simulink model "WaermepumpeGrundlageIch"  (R2013a)
settings: Solver=ode4  StartTime=0.0  StopTime=inf  RelTol=1e-3
libraries: Thermolib x74, simulink x2
(part 1 of 2)
settings Model: Creator=studi  LastModifiedBy=Admin
settings DataIOCC: SignalLoggingSaveFormat=ModelDataLogs
settings DebuggingCC: MultiTaskDSMMsg=warning  MultiTaskCondExecSysMsg=none  StrictBusMsg=None
settings RTWCC: IncludeERTFirstTime=on
settings GRTTargetCC: CodeReplacementLibrary=None  CPPClassGenCompliant=on

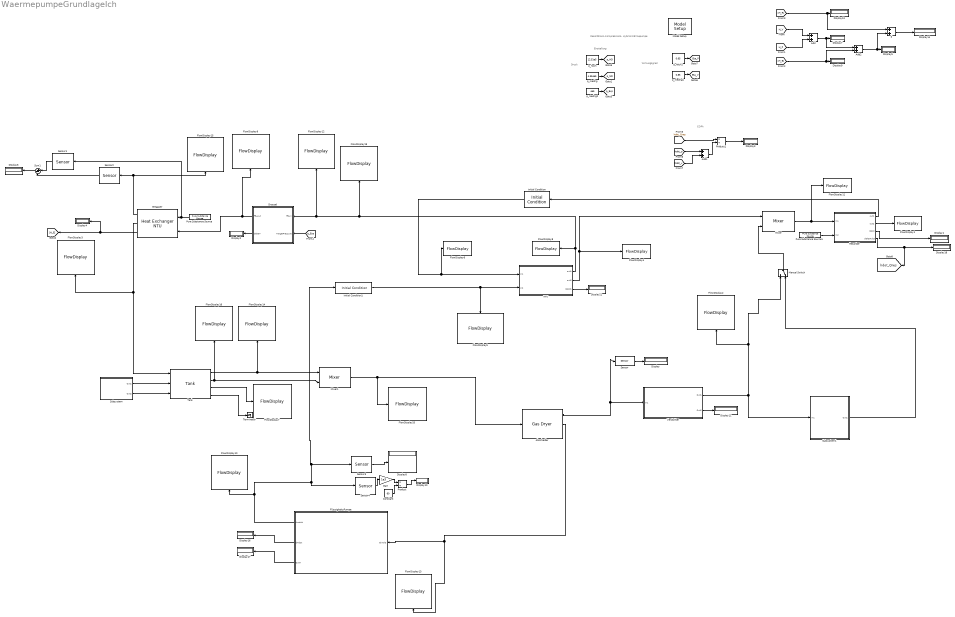
== system WaermepumpeGrundlageIch ==
  note: Resorbtions-Kompressions-
      | Hybrid-Wärmepumpe
  note: Einstellung
  note: Druck
  note: Wirkungsgrad
  note: COPh
  Abscheider : Thermolib/Components/Heat and Mass Transfer/Gas Dryer  Abscheid_eff=[0.4 1]  ndots=[0 5]  P_Loss=[0,1e3]  show_pf_ports=off  show_info_port=on  default_order_in_ports={'in','PFin'}  default_order_out_ports={'out','liquid','PFout','info'}
  Add : Sum
  Add1 : Sum
  Add2 : Sum
  Constant : Constant  Value=60
  Display{,1..11,13..14,16..18,21} (18 alike) : Display
  Drossel : Subsystem
      mask help: Jawooohl
      mask Help: Looking for help??
      mask Display:
      | fprintf('Isenthalp')
      | port_label('input', 1, 'in');
      | port_label('input', 2, 'p_target');
      | port_label('output', 1, 'out');
      | port_label('output', 2, '\Delta T','texmode','on');
  Entgaser : Thermolib/Components/Heat and Mass Transfer/Heat Exchanger NTU  selection=Counter Flow  show_UA_port=off  UA_Overall=3000  T_initial=273+20  A_env=1  T_env=273+25  k_env=0  p_loss_1=[0,1e3]  p_loss_2=[0,1e3]  thermal_mass=1  UA_flow1_mass1=0  UA_flow2_mass2=0  show_pf_ports=off  show_info_port=off  default_order_in_ports={'in1','in2','PFin1','PFin2'}  default_order_out_ports={'out1','out2','Qdot','PFout1','PFout2','info'}
  FlowDisplay1 : Thermolib/Sinks/FlowDisplay  bus_type=FlowBus  mdot=off kg/s  m_unit=mg  ndot=off mol/s  n_unit=mmol  temperature=on  T_unit=Celsius  pressure=on  p_unit=Pa  enthalpy=off  Hdot_unit=W  H_unit=mJ  entropy=off  Sdot_unit=W/K  S_unit=mJ/K  gibbs_energy=off  Gdot_unit=W  G_unit=mJ  heat_capacity=off  Cpdot_unit=W/K  Cp_unit=mJ/K  energy_content=off  U_unit=mW/K  vapor_fraction=off  molar_fraction=off  flag=0.8152
  FlowDisplay10 : Thermolib/Sinks/FlowDisplay  bus_type=FlowBus  mdot=off kg/s  m_unit=mg  ndot=on mol/s  n_unit=mmol  temperature=on  T_unit=Kelvin  pressure=on  p_unit=bar  enthalpy=on  Hdot_unit=W  H_unit=mJ  entropy=off  Sdot_unit=W/K  S_unit=mJ/K  gibbs_energy=off  Gdot_unit=W  G_unit=mJ  heat_capacity=off  Cpdot_unit=W/K  Cp_unit=mJ/K  energy_content=off  U_unit=mW/K  vapor_fraction=on  molar_fraction=on  flag=0.1812
  FlowDisplay11 : Thermolib/Sinks/FlowDisplay  bus_type=FlowBus  mdot=off kg/s  m_unit=mg  ndot=off mol/s  n_unit=mmol  temperature=on  T_unit=Celsius  pressure=on  p_unit=Pa  enthalpy=off  Hdot_unit=W  H_unit=mJ  entropy=off  Sdot_unit=W/K  S_unit=mJ/K  gibbs_energy=off  Gdot_unit=W  G_unit=mJ  heat_capacity=off  Cpdot_unit=W/K  Cp_unit=mJ/K  energy_content=off  U_unit=mW/K  vapor_fraction=off  molar_fraction=off  flag=0.1282
  FlowDisplay12 : Thermolib/Sinks/FlowDisplay  bus_type=FlowBus  mdot=off kg/s  m_unit=mg  ndot=off mol/s  n_unit=mmol  temperature=on  T_unit=Celsius  pressure=on  p_unit=bar  enthalpy=off  Hdot_unit=W  H_unit=mJ  entropy=off  Sdot_unit=W/K  S_unit=mJ/K  gibbs_energy=off  Gdot_unit=W  G_unit=mJ  heat_capacity=off  Cpdot_unit=W/K  Cp_unit=mJ/K  energy_content=off  U_unit=mW/K  vapor_fraction=off  molar_fraction=off  flag=0.5199
  FlowDisplay13 : Thermolib/Sinks/FlowDisplay  bus_type=FlowBus  mdot=off kg/s  m_unit=mg  ndot=on mol/s  n_unit=mmol  temperature=on  T_unit=Kelvin  pressure=on  p_unit=bar  enthalpy=on  Hdot_unit=W  H_unit=mJ  entropy=off  Sdot_unit=W/K  S_unit=mJ/K  gibbs_energy=off  Gdot_unit=W  G_unit=mJ  heat_capacity=off  Cpdot_unit=W/K  Cp_unit=mJ/K  energy_content=off  U_unit=mW/K  vapor_fraction=on  molar_fraction=on  flag=0.9645
  FlowDisplay14 : Thermolib/Sinks/FlowDisplay  bus_type=FlowBus  mdot=off kg/s  m_unit=mg  ndot=off mol/s  n_unit=mmol  temperature=on  T_unit=Celsius  pressure=on  p_unit=bar  enthalpy=off  Hdot_unit=W  H_unit=mJ  entropy=off  Sdot_unit=W/K  S_unit=mJ/K  gibbs_energy=off  Gdot_unit=W  G_unit=mJ  heat_capacity=off  Cpdot_unit=W/K  Cp_unit=mJ/K  energy_content=off  U_unit=mW/K  vapor_fraction=off  molar_fraction=off  flag=0.9654
  FlowDisplay15 : Thermolib/Sinks/FlowDisplay  bus_type=FlowBus  mdot=on kg/s  m_unit=mg  ndot=on mol/s  n_unit=mmol  temperature=on  T_unit=Kelvin  pressure=on  p_unit=bar  enthalpy=on  Hdot_unit=W  H_unit=mJ  entropy=off  Sdot_unit=W/K  S_unit=mJ/K  gibbs_energy=off  Gdot_unit=W  G_unit=mJ  heat_capacity=on  Cpdot_unit=W/K  Cp_unit=mJ/K  energy_content=off  U_unit=mW/K  vapor_fraction=on  molar_fraction=on  flag=0.8000
  FlowDisplay16 : Thermolib/Sinks/FlowDisplay  bus_type=FlowBus  mdot=off kg/s  m_unit=mg  ndot=off mol/s  n_unit=mmol  temperature=on  T_unit=Celsius  pressure=on  p_unit=bar  enthalpy=off  Hdot_unit=W  H_unit=mJ  entropy=off  Sdot_unit=W/K  S_unit=mJ/K  gibbs_energy=off  Gdot_unit=W  G_unit=mJ  heat_capacity=off  Cpdot_unit=W/K  Cp_unit=mJ/K  energy_content=off  U_unit=mW/K  vapor_fraction=off  molar_fraction=off  flag=0.3184
  FlowDisplay19 : Thermolib/Sinks/FlowDisplay  bus_type=FlowBus  mdot=off kg/s  m_unit=mg  ndot=on mol/s  n_unit=mmol  temperature=on  T_unit=Kelvin  pressure=on  p_unit=bar  enthalpy=on  Hdot_unit=W  H_unit=mJ  entropy=off  Sdot_unit=W/K  S_unit=mJ/K  gibbs_energy=off  Gdot_unit=W  G_unit=mJ  heat_capacity=off  Cpdot_unit=W/K  Cp_unit=mJ/K  energy_content=off  U_unit=mW/K  vapor_fraction=on  molar_fraction=on  flag=0.3878
  FlowDisplay2 : Thermolib/Sinks/FlowDisplay  bus_type=FlowBus  mdot=off kg/s  m_unit=mg  ndot=on mol/s  n_unit=mmol  temperature=on  T_unit=Celsius  pressure=on  p_unit=bar  enthalpy=on  Hdot_unit=W  H_unit=mJ  entropy=off  Sdot_unit=W/K  S_unit=mJ/K  gibbs_energy=off  Gdot_unit=W  G_unit=mJ  heat_capacity=off  Cpdot_unit=W/K  Cp_unit=mJ/K  energy_content=off  U_unit=mW/K  vapor_fraction=on  molar_fraction=on  flag=0.7145
  FlowDisplay20 : Thermolib/Sinks/FlowDisplay  bus_type=StateBus  mdot=on kg/s  m_unit=kg  ndot=off mol/s  n_unit=mol  temperature=on  T_unit=Celsius  pressure=on  p_unit=bar  enthalpy=on  Hdot_unit=W  H_unit=J  entropy=off  Sdot_unit=W/K  S_unit=mJ/K  gibbs_energy=off  Gdot_unit=W  G_unit=mJ  heat_capacity=off  Cpdot_unit=W/K  Cp_unit=mJ/K  energy_content=off  U_unit=mW/K  vapor_fraction=on  molar_fraction=on  flag=0.8658
  FlowDisplay3 : Thermolib/Sinks/FlowDisplay  bus_type=FlowBus  mdot=off kg/s  m_unit=mg  ndot=off mol/s  n_unit=mmol  temperature=on  T_unit=Celsius  pressure=on  p_unit=bar  enthalpy=off  Hdot_unit=W  H_unit=mJ  entropy=off  Sdot_unit=W/K  S_unit=mJ/K  gibbs_energy=off  Gdot_unit=W  G_unit=mJ  heat_capacity=off  Cpdot_unit=W/K  Cp_unit=mJ/K  energy_content=off  U_unit=mW/K  vapor_fraction=off  molar_fraction=off  flag=0.0870
  FlowDisplay4 : Thermolib/Sinks/FlowDisplay  bus_type=FlowBus  mdot=off kg/s  m_unit=mg  ndot=off mol/s  n_unit=mmol  temperature=on  T_unit=Kelvin  pressure=on  p_unit=Pa  enthalpy=off  Hdot_unit=W  H_unit=mJ  entropy=off  Sdot_unit=W/K  S_unit=mJ/K  gibbs_energy=off  Gdot_unit=W  G_unit=mJ  heat_capacity=off  Cpdot_unit=W/K  Cp_unit=mJ/K  energy_content=off  U_unit=mW/K  vapor_fraction=off  molar_fraction=off  flag=0.2788
  FlowDisplay5 : Thermolib/Sinks/FlowDisplay  bus_type=FlowBus  mdot=off kg/s  m_unit=mg  ndot=off mol/s  n_unit=mmol  temperature=on  T_unit=Kelvin  pressure=on  p_unit=Pa  enthalpy=off  Hdot_unit=W  H_unit=mJ  entropy=off  Sdot_unit=W/K  S_unit=mJ/K  gibbs_energy=off  Gdot_unit=W  G_unit=mJ  heat_capacity=off  Cpdot_unit=W/K  Cp_unit=mJ/K  energy_content=off  U_unit=mW/K  vapor_fraction=off  molar_fraction=off  flag=0.0144
  FlowDisplay6 : Thermolib/Sinks/FlowDisplay  bus_type=FlowBus  mdot=off kg/s  m_unit=mg  ndot=off mol/s  n_unit=mmol  temperature=on  T_unit=Kelvin  pressure=on  p_unit=Pa  enthalpy=off  Hdot_unit=W  H_unit=mJ  entropy=off  Sdot_unit=W/K  S_unit=mJ/K  gibbs_energy=off  Gdot_unit=W  G_unit=mJ  heat_capacity=off  Cpdot_unit=W/K  Cp_unit=mJ/K  energy_content=off  U_unit=mW/K  vapor_fraction=off  molar_fraction=off  flag=0.8314
  FlowDisplay7 : Thermolib/Sinks/FlowDisplay  bus_type=StateBus  mdot=on kg/s  m_unit=kg  ndot=off mol/s  n_unit=mol  temperature=on  T_unit=Celsius  pressure=on  p_unit=bar  enthalpy=on  Hdot_unit=W  H_unit=J  entropy=off  Sdot_unit=W/K  S_unit=mJ/K  gibbs_energy=off  Gdot_unit=W  G_unit=mJ  heat_capacity=off  Cpdot_unit=W/K  Cp_unit=mJ/K  energy_content=off  U_unit=mW/K  vapor_fraction=on  molar_fraction=on  flag=0.6126
  FlowDisplay8 : Thermolib/Sinks/FlowDisplay  bus_type=FlowBus  mdot=off kg/s  m_unit=mg  ndot=off mol/s  n_unit=mmol  temperature=on  T_unit=Kelvin  pressure=on  p_unit=Pa  enthalpy=off  Hdot_unit=W  H_unit=mJ  entropy=off  Sdot_unit=W/K  S_unit=mJ/K  gibbs_energy=off  Gdot_unit=W  G_unit=mJ  heat_capacity=off  Cpdot_unit=W/K  Cp_unit=mJ/K  energy_content=off  U_unit=mW/K  vapor_fraction=off  molar_fraction=off  flag=0.0312
  FlowDisplay9 : Thermolib/Sinks/FlowDisplay  bus_type=FlowBus  mdot=off kg/s  m_unit=mg  ndot=off mol/s  n_unit=mmol  temperature=on  T_unit=Celsius  pressure=on  p_unit=bar  enthalpy=off  Hdot_unit=W  H_unit=mJ  entropy=off  Sdot_unit=W/K  S_unit=mJ/K  gibbs_energy=off  Gdot_unit=W  G_unit=mJ  heat_capacity=off  Cpdot_unit=W/K  Cp_unit=mJ/K  energy_content=off  U_unit=mW/K  vapor_fraction=off  molar_fraction=off  flag=0.5216
  FlüssigkeitsPumpe : Subsystem
      mask Display:
      | path=pwd;
      | path_n=cat(2,pwd,'\Pumpe.PNG');
      | image(path_n);
      | port_label('input', 1, 'In');
      | port_label('output', 1, 'Out');
      | port_label('output', 3, 'Eta_p');
      | port_label('output', 2, 'dh');
  Gain : Gain  Gain=1e3
  IWU : Subsystem  mask(Heat Exchanger NTU){selection=Counter Flow, show_UA_port=off, UA_Overall=100, T_initial=273+20, A_env=1, T_env=273+20, k_env=0, p_loss_1=[0,1e1], p_loss_2=[0,1e1], thermal_mass=1, UA_flow1_mass1=0, UA_flow2_mass2=0, show_pf_ports=off, show_info_port=off, default_order_in_ports={'in1','in2','PFin1','PFin2'}, default_order_out_ports={'out1','out2','Qdot','PFout1','PFout2','info'}}
      mask prompts: selection "Flow direction:"; show_UA_port "Overall heat exchange coefficient from external"; UA_Overall "Coefficient of overall heat transfer rate [W/K]:"; T_initial "Initial temperature [K]:"; A_env "Total surface to environment  [m^2]:"; T_env "Environment temperature [K]:"; k_env "Coefficient for calculating heat exchange with the environment [W / m2 K]:"; p_loss_1 "Pressure loss factor [Pa/(g/s) 2] and minimum downstream pressure [Pa] for first flow:"; p_loss_2 "Pressure loss factor [Pa/(g/s) 2] and minimum downstream pressure [Pa] for second flow:"; thermal_mass "Thermal mass of the heat exchanger [Joules/K]:"; UA_flow1_mass1 "Coefficient of heat transfer rate from flow 1 to thermal mass 1 [W/K]"; UA_flow2_mass2 "Coefficient of heat transfer rate from flow 2 to thermal mass 2 [W/K]"; show_pf_ports "Show pressure feedback ports"; show_info_port "Show info port"
      mask help:
      | The Heat Exchanger block calculates the change of state of two media caused by indirect heat exchange. Three types of exchange are supported: counter flow, parallel flow and cross flow.
      |
      | The NTU-Method (number of transfer unit), used to model the heat exchanger, calculates the maximum possible heat transfer between the two flows. The actual heat transfer rate can be determined by calculating the effectiveness, which is the actual heat transfer divided by the maximum possible heat transfer.
      |
      | To model the thermal dynamics the input flows are passed through two thermal mass elements.
      mask init:
      | set_param(gcb, 'MaskSelfModifiable', 'on');
      | 
      | if selection==3
      |   icon = imread('heat_ex_pa.tif','tif');
      | end
      | if selection==1
      |   icon = imread('heat_ex_co.tif','tif');
      | end
      | if selection==2
      |   icon = imread('heat_ex_cr.tif','tif');
      | end
      | 
      | blk = gcb;
      | ioc = zeros(1,6);
      | 
      | ioc(1) = th_ShowPorts(blk,'PFin1','show_pf_ports','in','built-in/Constant',{'Value','0'});
      | ioc(2) = th_ShowPorts(blk,'PFin2','show_pf_ports','in','built-in/Constant',{'Value','0'});
      | ioc(3) = th_ShowPorts(blk,'UA','show_UA_port','in','built-in/Constant',{'Value','UA_Overall'});
      | ioc(4) = th_ShowPorts(blk,'PFout1','show_pf_ports','out','built-in/Terminator');
      | ioc(5) = th_ShowPorts(blk,'PFout2','show_pf_ports','out','built-in/Terminator');
      | ioc(6) = th_ShowPorts(blk,'info','show_info_port','out','built-in/Terminator');
      | 
      | if any(ioc)
      | 	base_draw_cmd = 'image(icon,[0.2,0.1,0.6,0.8])';
      | 	th_AddPortsToDrawingCmd(blk,base_draw_cmd)
      | end
      mask Help: eval('th_StartBlockHelp(gcb)');
      mask TypeOptions selection: Counter Flow | Cross Flow | Parallel Flow
      mask Callback show_UA_port:
      | a = {'on','on','on','on','on','on','on','on','on','on','on','on','on','on','off','off'};
      | b = {'on','on','off','on','on','on','on','on','on','on','on','on','on','on','off','off'};
      | 
      | 
      | 
      | switch get_param(gcb, 'show_UA_port')
      |     case 'on'
      |         set_param(gcb,'MaskVisibilities',	[b] );
      |     case 'off'
      |         set_param(gcb,'MaskVisibilities',	[a]);
      | end
      mask Display:
      | image(icon,[0.2,0.1,0.6,0.8])
      | port_label('output',1,'out1')
      | port_label('output',2,'out2')
      | port_label('output',3,'Qdot')
      | port_label('input',1,'in1')
      | port_label('input',2,'in2')
  Initial Condition : Thermolib/Miscellaneous/Initial Condition  disp_str=fprintf('Initial conditions:\n T = 298.15 [K]\np = 100000 [Pa]')  T=298.15 C  T_in=25  p=100000 bar  p_in=1  psi=[0.3 0.7]  species_local={'H2O', 'NH3'}  psi_local=[0.3 0.7]  use_fb=on  ndot=1 mol/s  ndot_in=0  switch_flow_type=1  flow_type=Molar Flow  Hdot=-117669.870695777  Sdot=156.374582351195  Gdot=-164292.952423785  Cpdot=48.0782778924394  x=[0.0658877601640708;0.956663479644059]  show_pf_ports=off  default_order_in_ports=off  default_order_out_ports=off
  Initial Condition1 : Thermolib/Miscellaneous/Initial Condition  disp_str=fprintf('Initial conditions:\n T = 298.15 [K]\np = 100000 [Pa]')  T=298.15 C  T_in=25  p=100000 bar  p_in=1  psi=[0.3 0.7]  species_local={'H2O', 'NH3'}  psi_local=[0.3 0.7]  use_fb=on  ndot=1 mol/s  ndot_in=0  switch_flow_type=1  flow_type=Molar Flow  Hdot=-117669.870695777  Sdot=156.374582351195  Gdot=-164292.952423785  Cpdot=48.0782778924394  x=[0.0658877601640708;0.956663479644059]  show_pf_ports=off  default_order_in_ports=off  default_order_out_ports=off
  Manual Switch : ManualSwitch  CurrentSetting=0
  Mixer : Thermolib/Components/Hydraulic/Mixer  Mode=mixer  P_Loss=[0,0.01e5]  p_out_method=p_out = weighted_mean(p1_in;p2_in)  default_order_in_ports={'in1','in2','ratio','PFin'}  default_order_out_ports={'out','in2 ','PFout1','PFout2','info'}  show_pf_ports=off  show_info_port=off
  Mixer1 : Thermolib/Components/Hydraulic/Mixer  Mode=mixer  P_Loss=[0,0.01e5]  p_out_method=p_out = weighted_mean(p1_in;p2_in)  default_order_in_ports={'in1','in2','ratio','PFin'}  default_order_out_ports={'out','in2 ','PFout1','PFout2','info'}  show_pf_ports=off  show_info_port=off
  Model Setup : Thermolib/Setup/Model Setup  starttime=10  endtime=20  loadWS=on  loadWSCommand=fc_LoadWorkspace  media_file=ChemicalMediaData.mat  constants_file=Constants.mat  species_reduced={'H2O', 'NH3'}  load_model_command=load ComponentData.mat  gas_eos_method=1  gas_mixing_rule=0  species_allow_liquid=[1 1]  species_allow_vapor=[1 1]  last_saved_thermolib_version=5.1.2.5490  liquid_eos_method=1  density_calculation_mode=0
  Product : Product  Inputs=*/
  Product1 : Product  Inputs=*/
  Pure Substance Source : Thermolib/Sources/Pure Substance Source  disp_str=fprintf('H2O Mass flow')  flow_type=Mass flow  switch_flow_type=3  ndot=1002 kg/s  ndot_in=1.002  T=313.15 K  T_in=273.15+40  p=100000 Pa  p_in=1e+5  T_p_x_switch=2  x=1e-005  species_local={'H2O'}  psi_local=1  psi=[1 0]
  Pure Substance Source1 : Thermolib/Sources/Pure Substance Source  disp_str=fprintf('H2O Mass flow')  flow_type=Mass flow  switch_flow_type=3  ndot=1000 kg/s  ndot_in=1  T=313.15 K  T_in=273.15+40  p=100000 Pa  p_in=1e+5  T_p_x_switch=2  x=1e-005  species_local={'H2O'}  psi_local=1  psi=[1 0]
  Resorber : Subsystem  AncestorBlock=Thermolib/Components/Heat and Mass Transfer/Heat Exchanger NTU  mask(Heat Exchanger NTU){selection=Counter Flow, show_UA_port=off, UA_Overall=3000, T_initial=273+20, A_env=0, T_env=273+20, k_env=0, p_loss_1=[0,1e3], p_loss_2=[0,1e3], thermal_mass=0.1, UA_flow1_mass1=0, UA_flow2_mass2=0, show_pf_ports=off, show_info_port=off, default_order_in_ports={'in1','in2','PFin1','PFin2'}, default_order_out_ports={'out1','out2','Qdot','PFout1','PFout2','info'}}
      mask prompts: selection "Flow direction:"; show_UA_port "Overall heat exchange coefficient from external"; UA_Overall "Coefficient of overall heat transfer rate [W/K]:"; T_initial "Initial temperature [K]:"; A_env "Total surface to environment  [m^2]:"; T_env "Environment temperature [K]:"; k_env "Coefficient for calculating heat exchange with the environment [W / m2 K]:"; p_loss_1 "Pressure loss factor [Pa/(g/s) 2] and minimum downstream pressure [Pa] for first flow:"; p_loss_2 "Pressure loss factor [Pa/(g/s) 2] and minimum downstream pressure [Pa] for second flow:"; thermal_mass "Thermal mass of the heat exchanger [Joules/K]:"; UA_flow1_mass1 "Coefficient of heat transfer rate from flow 1 to thermal mass 1 [W/K]"; UA_flow2_mass2 "Coefficient of heat transfer rate from flow 2 to thermal mass 2 [W/K]"; show_pf_ports "Show pressure feedback ports"; show_info_port "Show info port"
      mask help:
      | The Heat Exchanger block calculates the change of state of two media caused by indirect heat exchange. Three types of exchange are supported: counter flow, parallel flow and cross flow.
      |
      | The NTU-Method (number of transfer unit), used to model the heat exchanger, calculates the maximum possible heat transfer between the two flows. The actual heat transfer rate can be determined by calculating the effectiveness, which is the actual heat transfer divided by the maximum possible heat transfer.
      |
      | To model the thermal dynamics the input flows are passed through two thermal mass elements.
      mask init: same as WaermepumpeGrundlageIch/IWU
      mask Help: eval('th_StartBlockHelp(gcb)');
      mask TypeOptions selection: Counter Flow | Cross Flow | Parallel Flow
      mask Callback show_UA_port:
      | a = {'on','on','on','on','on','on','on','on','on','on','on','on','on','on','off','off'};
      | b = {'on','on','off','on','on','on','on','on','on','on','on','on','on','on','off','off'};
      | 
      | 
      | 
      | switch get_param(gcb, 'show_UA_port')
      |     case 'on'
      |         set_param(gcb,'MaskVisibilities',	[b] );
      |     case 'off'
      |         set_param(gcb,'MaskVisibilities',	[a]);
      | end
      mask Display:
      | image(icon,[0.2,0.1,0.6,0.8])
      | port_label('output',1,'out1')
      | port_label('output',2,'out2')
      | port_label('output',3,'Qdot')
      | port_label('output',4,'deltaHdot')
      | port_label('input',1,'in1')
      | port_label('input',2,'in2')
  S : Sum
  Sensor : Thermolib/Miscellaneous/Sensor  lst_physical_value=vdot_gas measured in m^3/h;  mult_fac=3600  add_fac=0  selected_signals=14
  Sensor1 : Thermolib/Miscellaneous/Sensor  lst_physical_value=Hdot measured in W;  mult_fac=1  add_fac=0  selected_signals=4
  Sensor2 : Thermolib/Miscellaneous/Sensor  lst_physical_value=Hdot measured in W;  mult_fac=1  add_fac=0  selected_signals=4
  Sensor3 : Thermolib/Miscellaneous/Sensor  lst_physical_value=vdot_gas measured in m^3/h;vdot_liquid measured in m^3/h;mdot measured in kg/s;psi H2O measured in -;  mult_fac=[3600 3600 0.001 1]  add_fac=[0 0 0 0]  selected_signals=[14 16 13 11]
  Sensor4 : Thermolib/Miscellaneous/Sensor  lst_physical_value=vdot_liquid measured in m^3/h;  mult_fac=3600  add_fac=0  selected_signals=16
  Subsystem : Subsystem  mask{m=0, a1=0, a2=0}
      mask prompts: m "Massenstrom"; a1 "Wasser Anteil"; a2 "Ammoniak Anteil"
      mask Display: fprintf('Massenstromregler')
  Subsystem1 : Subsystem
      mask Display:
      | path=pwd;
      | path_n=cat(2,pwd,'\Abscheider.png');
      | image(path_n);
  Sum1 : Sum  Inputs=|+-
  Tank : Thermolib/Components/Tanks/Tank  Volume=0.1  T_init=273+25  p_init=4e5  psi_init=[0.3 0.7]  p_min=1e4  mdot_out_method1=m.out = external  mdot_out_method2=m.out = external  species_local={'H2O', 'NH3'}  psi_local=[0.3 0.7]  x_init=0.3  mdot_out_pf_max=1000  mdot_out_pf_initial=1  mdot_out_pf_relaxation=0.3  show_pfout1_port=off  show_pfout2_port=off  Generic_Tank_radiobutton=off  Adiabatic_Tank_radiobutton=on  Isothermal_Tank_radiobutton=off  show_in1_port=on  show_in2_port=off  show_out1_port=on  show_out2_port=on  show_mdot_out1_port=on  show_mdot_out2_port=on  show_pfin1_port=off  show_pfin2_port=off  default_order_in_ports={'in1','in2','mdot_out1','mdot_out2','Qdot','PFin1','PFin2'}  default_order_out_ports={'out1','out2','state',' Qdot','PFout1','PFout2','info'}  T_p_x_switch=3  position_out1=1  position_out2=0  show_info_port=on
  Terminator : Terminator
  Verdichter : Subsystem  Description=Verdichter (Selbstgemacht)  mask(Verdichter Selfmade){}
      mask help: Polytrop
      mask Help: Frag Anton
      mask Display:
      | path=pwd;
      | path_n=cat(2,pwd,'\Verdichter.PNG');
      | image(path_n);
      | port_label('input', 1, 'In');
      | port_label('output', 1, 'Out');
      | port_label('output', 2,'\Delta Hdot','texmode','on');
  p_hoch : Constant  Value=12.51e5
  p_hoch1 : Constant  Value=0.65
  p_niedrig : Constant  Value=4.354e5
  p_niedrig1 : Constant  Value=0.85
  p_niedrig2 : Constant  Value=4e5
  tag scope: Eta_P=global, Eta_V=global, hdot_Qres=global, p_Exp=global, p_HD=global, p_ND=global
  wires:
  Abscheider/2 -> FlowDisplay13/1, FlüssigkeitsPumpe/1(Eintritt)
  Pure Substance Source/1 -> Sensor1/1, Entgaser/1
  [p_Exp] -> Drossel/2(TargetPressure)
  Resorber/2(out2) -> FlowDisplay1/1
  Resorber/3(Qdot) -> Display1/1
  Entgaser/3 -> Display4/1, [H_E]
  Drossel/1(FB_out) -> FlowDisplay9/1, Entgaser/2
  Drossel/2(deltaT) -> Display2/1
  [H_V] -> Add/1
  [H_P] -> Add/2
  Add/1 -> Add2/1, Display7/1
  [H_E] -> Add2/2, Display9/1
  Resorber/1(out1) -> Initial Condition/1
  Mixer/1 -> FlowDisplay11/1, Resorber/1(in1)
  [H_R] -> S/1, Display13/1
  Add2/1 -> S/2, Display5/1
  S/1 -> Display14/1
  Tank/1 -> FlowDisplay14/1, Mixer1/1
  Tank/2 -> Mixer1/2, FlowDisplay16/1
  p_hoch/1 -> [p_HD]
  p_niedrig/1 -> [p_ND]
  p_hoch1/1 -> [Eta_P]
  p_niedrig1/1 -> [Eta_V]
  Entgaser/2 -> FlowDisplay3/1, Tank/1
  Tank/3 -> FlowDisplay7/1
  IWU/2(out2) -> FlowDisplay4/1, Mixer/1
  IWU/1(out1) -> Drossel/1(FB_in), FlowDisplay12/1, FlowDisplay19/1, FlowDisplay8/1
  Initial Condition/1 -> FlowDisplay6/1, IWU/1(in1)
  IWU/3(Qdot1) -> Display21/1
  Tank/4 -> Terminator/1
  ? -> ?
  Abscheider/1 -> Sensor/1, Verdichter/1(In1)
  FlüssigkeitsPumpe/1("Austritt ") -> FlowDisplay10/1, Initial Condition1/1, Sensor3/1, Sensor4/1
  FlüssigkeitsPumpe/2("dHdot ") -> Display16/1
  FlüssigkeitsPumpe/3(Out4) -> Display17/1
  Initial Condition1/1 -> FlowDisplay5/1, IWU/2(in2)
  Sensor/1 -> Display/1
  Mixer1/1 -> FlowDisplay20/1, Abscheider/1
  Sensor3/1 -> Display8/1
  Product/1 -> Display10/1
  Constant/1 -> Product/2
  Sensor4/1 -> Gain/1
  Gain/1 -> Product/1
  Pure Substance Source1/1 -> Resorber/2(in2)
  Entgaser/1 -> Sensor2/1, FlowDisplay15/1
  p_niedrig2/1 -> [p_Exp]
  Sensor1/1 -> Sum1/1
  Sensor2/1 -> Sum1/2
  Sum1/1 -> Display6/1
  Verdichter/2(Out2) -> Display11/1
  Resorber/4(deltaHdot) -> [hdot_Qres], Display18/1
  Subsystem/1(Out1) -> Tank/2
  Subsystem/2(Out2) -> Tank/3
  [hdot_Qres] -> Product1/1
  [hdot_p] -> Add1/1
  [hdot_v] -> Add1/2
  Add1/1 -> Product1/2
  Product1/1 -> Display3/1
  Manual Switch/1 -> Mixer/2
  Verdichter/1(Out1) -> Subsystem1/1(In1), FlowDisplay2/1, Manual Switch/1
  Subsystem1/1(Out1) -> Manual Switch/2

== system WaermepumpeGrundlageIch/Drossel ==
  FB_in : Inport
  TargetPressure : Inport  Port=2
  Bus Assignment3 : BusAssignment  AssignedSignals=p
  Bus Selector5 : BusSelector  OutputSignals=p
  H-p-State : Thermolib/Thermodynamic States and Properties/H-p-State with Heat Exchange  k=0  A_total=0  T_env=273+20  relaxation_factor=0.01  conv_limit=0.1  hm_conv_limit=TH_THERM_H_P_STATE_HM_CONV_LIMIT  n_iteration=TH_THERM_H_P_STATE_NUM_ITER_MAX  T_initial=273+20  H_initial=0  ndot_zero_eps=1e-9
  MinMax : MinMax  Inputs=2
  Subtract : Sum  Inputs=+-
  T1 : BusSelector  OutputSignals=T
  T2 : BusSelector  OutputSignals=T
  Terminator3 : Terminator
  Terminator4 : Terminator
  FB_out : Outport
  deltaT : Outport  Port=2
  wires:
  H-p-State/1 -> T2/1, FB_out/1
  H-p-State/3 -> Terminator4/1
  H-p-State/2 -> Terminator3/1
  Bus Assignment3/1 -> H-p-State/1
  FB_in/1 -> T1/1, Bus Assignment3/1, Bus Selector5/1
  Bus Selector5/1 -> MinMax/1  "<p>"
  TargetPressure/1 -> MinMax/2
  MinMax/1 -> Bus Assignment3/2
  T1/1 -> Subtract/1  "<T>"
  T2/1 -> Subtract/2  "<T>"
  Subtract/1 -> deltaT/1

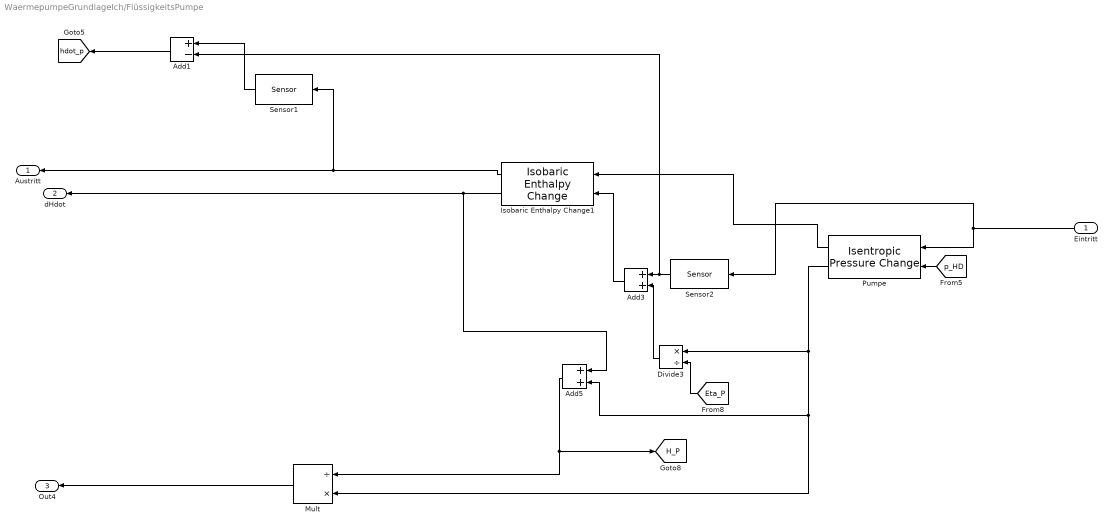
== system WaermepumpeGrundlageIch/FlüssigkeitsPumpe ==
  Eintritt : Inport
  Add1 : Sum  Inputs=+-
  Add3 : Sum
  Add5 : Sum
  Divide3 : Product  Inputs=*/
  Isobaric Enthalpy Change1 : Thermolib/Thermodynamic State Changes/Isobaric Enthalpy Change
  Mult : Product  Inputs=/*
  Pumpe : Thermolib/Thermodynamic State Changes/Isentropic Pressure Change
  Sensor1 : Thermolib/Miscellaneous/Sensor  lst_physical_value=Hdot measured in W;  mult_fac=1  add_fac=0  selected_signals=4
  Sensor2 : Thermolib/Miscellaneous/Sensor  lst_physical_value=Hdot measured in W;  mult_fac=1  add_fac=0  selected_signals=4
  "Austritt " : Outport
  "dHdot " : Outport  Port=2
  Out4 : Outport  Port=3
  tag scope: H_P=global, hdot_p=global
  wires:
  Eintritt/1 -> Pumpe/1, Sensor2/1
  Pumpe/2 -> Mult/2, Add5/2, Divide3/1
  [p_HD] -> Pumpe/2
  Pumpe/1 -> Isobaric Enthalpy Change1/1
  [Eta_P] -> Divide3/2
  Sensor2/1 -> Add1/2, Add3/1
  Divide3/1 -> Add3/2
  Add3/1 -> Isobaric Enthalpy Change1/2
  Isobaric Enthalpy Change1/2 -> Add5/1, "dHdot "/1
  Mult/1 -> Out4/1
  Add5/1 -> Mult/1, [H_P]
  Isobaric Enthalpy Change1/1 -> Sensor1/1, "Austritt "/1
  Add1/1 -> [hdot_p]
  Sensor1/1 -> Add1/1

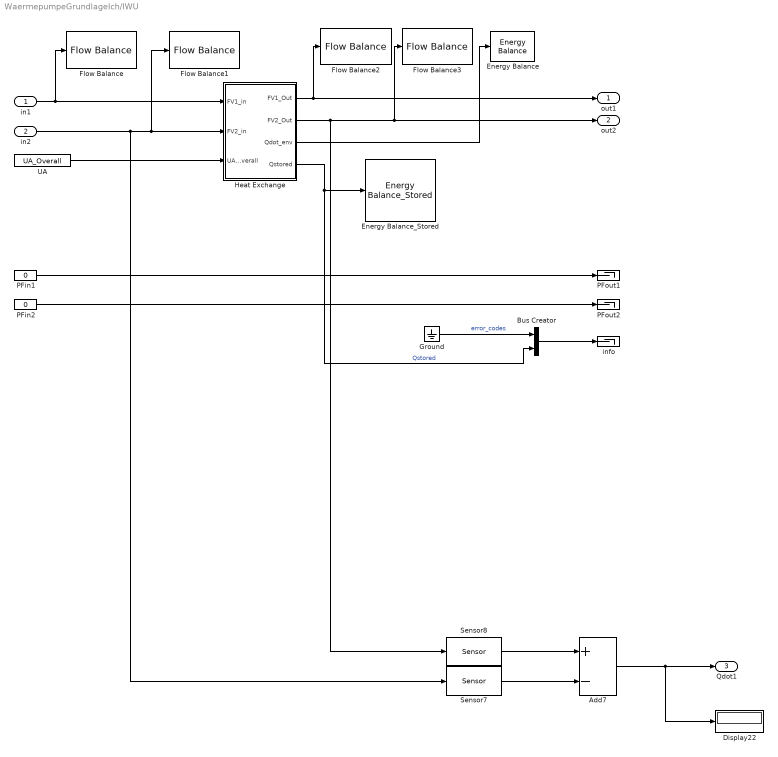
== system WaermepumpeGrundlageIch/IWU ==
  in1 : Inport
  in2 : Inport  Port=2
  Add7 : Sum  Inputs=+-
  Bus Creator : BusCreator  Inputs=2
  Display22 : Display
  Energy Balance : Thermolib/Balance/Energy Balance  asklabel=Use name of parent system  mainlabel=Thermolib/Components/Heat and Mass Transfer/Heat Exchanger NTU  label='Qdot environment'
  Energy Balance_Stored : Thermolib/Balance/Energy Balance_Stored  asklabel=Use name of parent system  mainlabel=Thermolib/Components/Heat and Mass Transfer/Heat Exchanger NTU  label='thermal mass energy'
  Flow Balance : Thermolib/Balance/Flow Balance  asklabel=Use name of parent system  mainlabel='Name here'  direction=in  label='In1'
  Flow Balance1 : Thermolib/Balance/Flow Balance  asklabel=Use name of parent system  mainlabel='Name here'  direction=in  label='in2'
  Flow Balance2 : Thermolib/Balance/Flow Balance  asklabel=Use name of parent system  mainlabel='Name here'  direction=out  label='out1'
  Flow Balance3 : Thermolib/Balance/Flow Balance  asklabel=Use name of parent system  mainlabel='Name here'  direction=out  label='out2'
  Ground : Ground
  Heat Exchange : Subsystem  TreatAsAtomicUnit=on
  PFin1 : Constant  Value=0
  PFin2 : Constant  Value=0
  PFout1 : Terminator
  PFout2 : Terminator
  Sensor7 : Thermolib/Miscellaneous/Sensor  lst_physical_value=Hdot measured in W;  mult_fac=1  add_fac=0  selected_signals=4
  Sensor8 : Thermolib/Miscellaneous/Sensor  lst_physical_value=Hdot measured in W;  mult_fac=1  add_fac=0  selected_signals=4
  UA : Constant  Value=UA_Overall
  info : Terminator
  out1 : Outport
  out2 : Outport  Port=2
  Qdot1 : Outport  Port=3
  wires:
  Ground/1 -> Bus Creator/1  "error_codes"
  Bus Creator/1 -> info/1
  Heat Exchange/4(Qstored) -> Bus Creator/2, Energy Balance_Stored/1  "Qstored"
  Heat Exchange/3(Qdot_env) -> Energy Balance/1
  Heat Exchange/1(FV1_Out) -> Flow Balance2/1, out1/1
  in1/1 -> Heat Exchange/1(FV1_in), Flow Balance/1
  PFin1/1 -> PFout1/1
  PFin2/1 -> PFout2/1
  UA/1 -> Heat Exchange/3(UA_overall)
  Heat Exchange/2(FV2_Out) -> Sensor8/1, Flow Balance3/1, out2/1
  in2/1 -> Sensor7/1, Flow Balance1/1, Heat Exchange/2(FV2_in)
  Sensor7/1 -> Add7/2
  Sensor8/1 -> Add7/1
  Add7/1 -> Qdot1/1, Display22/1

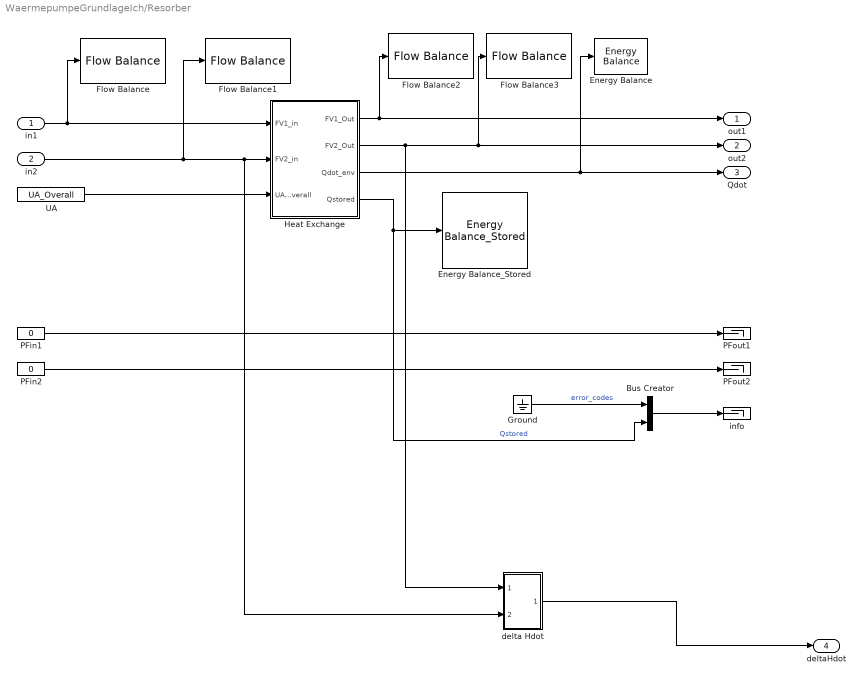
== system WaermepumpeGrundlageIch/Resorber ==
  in1 : Inport
  in2 : Inport  Port=2
  Bus Creator : BusCreator  Inputs=2
  Energy Balance : Thermolib/Balance/Energy Balance  asklabel=Use name of parent system  mainlabel=Thermolib/Components/Heat and Mass Transfer/Heat Exchanger NTU  label='Qdot environment'
  Energy Balance_Stored : Thermolib/Balance/Energy Balance_Stored  asklabel=Use name of parent system  mainlabel=Thermolib/Components/Heat and Mass Transfer/Heat Exchanger NTU  label='thermal mass energy'
  Flow Balance : Thermolib/Balance/Flow Balance  asklabel=Use name of parent system  mainlabel='Name here'  direction=in  label='In1'
  Flow Balance1 : Thermolib/Balance/Flow Balance  asklabel=Use name of parent system  mainlabel='Name here'  direction=in  label='in2'
  Flow Balance2 : Thermolib/Balance/Flow Balance  asklabel=Use name of parent system  mainlabel='Name here'  direction=out  label='out1'
  Flow Balance3 : Thermolib/Balance/Flow Balance  asklabel=Use name of parent system  mainlabel='Name here'  direction=out  label='out2'
  Ground : Ground
  Heat Exchange : Subsystem  TreatAsAtomicUnit=on
  PFin1 : Constant  Value=0
  PFin2 : Constant  Value=0
  PFout1 : Terminator
  PFout2 : Terminator
  UA : Constant  Value=UA_Overall
  delta Hdot : Subsystem
  info : Terminator
  out1 : Outport
  out2 : Outport  Port=2
  Qdot : Outport  Port=3
  deltaHdot : Outport  Port=4
  wires:
  UA/1 -> Heat Exchange/3(UA_overall)
  PFin2/1 -> PFout2/1
  PFin1/1 -> PFout1/1
  in1/1 -> Flow Balance/1, Heat Exchange/1(FV1_in)
  Heat Exchange/1(FV1_Out) -> out1/1, Flow Balance2/1
  Heat Exchange/3(Qdot_env) -> Qdot/1, Energy Balance/1
  Heat Exchange/4(Qstored) -> Energy Balance_Stored/1, Bus Creator/2  "Qstored"
  Bus Creator/1 -> info/1
  Ground/1 -> Bus Creator/1  "error_codes"
  Heat Exchange/2(FV2_Out) -> delta Hdot/1(In1), out2/1, Flow Balance3/1
  in2/1 -> delta Hdot/2(In2), Heat Exchange/2(FV2_in), Flow Balance1/1
  delta Hdot/1(Out1) -> deltaHdot/1

== system WaermepumpeGrundlageIch/Subsystem ==
  2 : Constant  Value=0.7
  3 : Constant  Value=0.3
  4 : Constant  Value=164.8
  Product : Product
  Product1 : Product
  Out1 : Outport
  Out2 : Outport  Port=2
  wires:
  3/1 -> Product1/2
  Product1/1 -> Out2/1
  2/1 -> Product/2
  4/1 -> Product1/1, Product/1
  Product/1 -> Out1/1

== system WaermepumpeGrundlageIch/Subsystem1 ==
  note: Enthalpieänderung durch Ölkühlung
      | -massenstrom des öls ist 10% von gasmassenstrom
      | - cp konstant aus EES
      | Taustritt heizung ist = Gastemperatur
  In1 : Inport
  Constant1 : Constant  Value=2100
  Constant2 : Constant  Value=273.15+60
  Display12 : Display
  Display15 : Display
  Display19 : Display
  Gain1 : Gain  Gain=0.1
  Isobaric Enthalpy Change : Thermolib/Thermodynamic State Changes/Isobaric Enthalpy Change
  Product2 : Product
  Product3 : Product
  Sensor5 : Thermolib/Miscellaneous/Sensor  lst_physical_value=mdot measured in kg/s;  mult_fac=0.001  add_fac=0  selected_signals=13
  Sensor6 : Thermolib/Miscellaneous/Sensor  lst_physical_value=T measured in K;  mult_fac=1  add_fac=0  selected_signals=2
  Sensor7 : Thermolib/Miscellaneous/Sensor  lst_physical_value=Hdot measured in W;  mult_fac=1  add_fac=0  selected_signals=4
  Sum : Sum  Inputs=-+
  Sum2 : Sum  Inputs=+-
  Out1 : Outport
  wires:
  Sensor7/1 -> Display19/1, Sum2/1
  Isobaric Enthalpy Change/2 -> Display15/1
  Sum2/1 -> Isobaric Enthalpy Change/2
  Isobaric Enthalpy Change/1 -> Display12/1, Out1/1
  Product3/1 -> Sum2/2
  Sensor5/1 -> Gain1/1
  Sensor6/1 -> Sum/2
  Constant1/1 -> Product2/1
  Gain1/1 -> Product3/2
  Sum/1 -> Product2/2
  Constant2/1 -> Sum/1
  Product2/1 -> Product3/1
  In1/1 -> Sensor5/1, Sensor6/1, Sensor7/1, Isobaric Enthalpy Change/1

== system WaermepumpeGrundlageIch/Verdichter ==
  In1 : Inport
  Display8 : Display
  Isobaric Enthalpy Change : Thermolib/Thermodynamic State Changes/Isobaric Enthalpy Change
  Sensor1 : Thermolib/Miscellaneous/Sensor  lst_physical_value=Hdot measured in W;  mult_fac=1  add_fac=0  selected_signals=4
  Sensor4 : Thermolib/Miscellaneous/Sensor  lst_physical_value=Hdot measured in W;  mult_fac=1  add_fac=0  selected_signals=4
  Subsystem1 : Subsystem
  Subtract : Sum  Inputs=+-
  Verdichter : Thermolib/Thermodynamic State Changes/Isentropic Pressure Change
  Out1 : Outport
  Out2 : Outport  Port=2
  tag scope: hdot_v=global
  wires:
  In1/1 -> Verdichter/1, Sensor4/1
  Verdichter/1 -> Isobaric Enthalpy Change/1
  [p_HD] -> Verdichter/2
  Verdichter/2 -> Subsystem1/2(In2), Display8/1
  Isobaric Enthalpy Change/2 -> Subsystem1/1(In1)
  [Eta_V] -> Subsystem1/3(In4)
  Sensor4/1 -> Subtract/2, Subsystem1/4(In5)
  Subsystem1/1(Out1) -> Isobaric Enthalpy Change/2
  Isobaric Enthalpy Change/1 -> Sensor1/1, Out1/1
  Sensor1/1 -> Subtract/1
  Subtract/1 -> [hdot_v], Out2/1

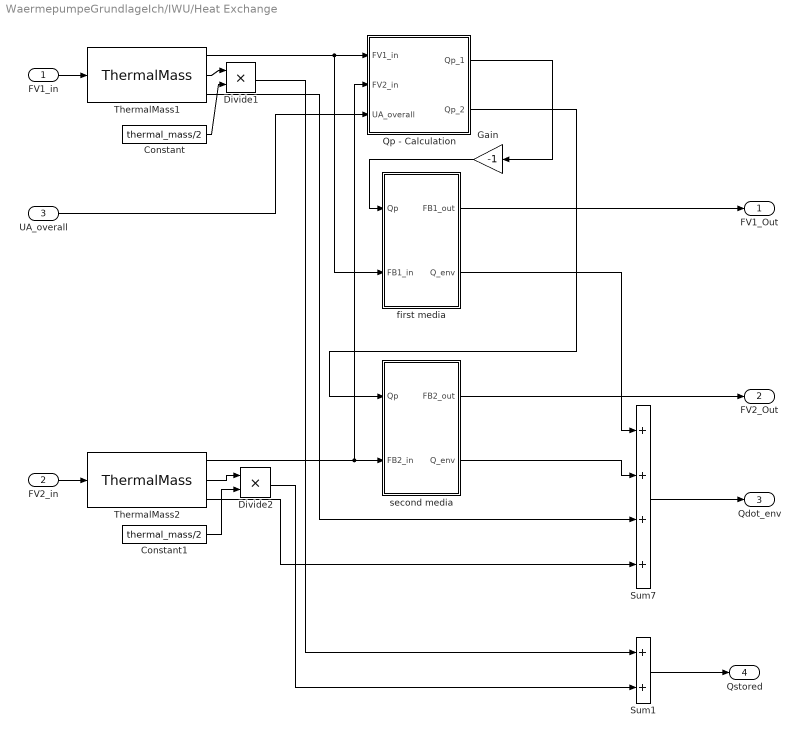
== system WaermepumpeGrundlageIch/IWU/Heat Exchange ==
  FV1_in : Inport
  FV2_in : Inport  Port=2
  UA_overall : Inport  Port=3
  Constant : Constant  Value=thermal_mass/2
  Constant1 : Constant  Value=thermal_mass/2
  Divide1 : Product  Inputs=**
  Divide2 : Product  Inputs=**
  Gain : Gain  Gain=-1  SaturateOnIntegerOverflow=on  OutDataTypeStr=Inherit: Same as input  ParamDataTypeStr=Inherit: Same as input
  Qp - Calculation : Subsystem
  Sum1 : Sum  Inputs=2  SaturateOnIntegerOverflow=on  InputSameDT=on  OutDataTypeStr=Inherit: Same as first input
  Sum7 : Sum  Inputs=4  SaturateOnIntegerOverflow=on  InputSameDT=on  OutDataTypeStr=Inherit: Same as first input
  ThermalMass1 : Thermolib/Components/Heat and Mass Transfer/Thermal Mass/ThermalMass  A_env=A_env/4  k_env=k_env  T_env=T_env  p_loss=p_loss_1  thermal_mass=thermal_mass/2  T_initial=T_initial  UA_flow_mass=UA_flow1_mass1
  ThermalMass2 : Thermolib/Components/Heat and Mass Transfer/Thermal Mass/ThermalMass  A_env=A_env/4  k_env=k_env  T_env=T_env  p_loss=p_loss_2  thermal_mass=thermal_mass/2  T_initial=T_initial  UA_flow_mass=UA_flow2_mass2
  first media : Subsystem
  second media : Subsystem
  FV1_Out : Outport  InitialOutput=[0]
  FV2_Out : Outport  Port=2  InitialOutput=[0]
  Qdot_env : Outport  Port=3  InitialOutput=[0]
  Qstored : Outport  Port=4  InitialOutput=[0]
  wires:
  Divide2/1 -> Sum1/2
  Constant1/1 -> Divide2/2
  Constant/1 -> Divide1/2
  Divide1/1 -> Sum1/1
  Sum1/1 -> Qstored/1
  FV2_in/1 -> ThermalMass2/1
  FV1_in/1 -> ThermalMass1/1
  ThermalMass1/3 -> Sum7/3
  ThermalMass2/3 -> Sum7/4
  ThermalMass2/1 -> second media/2(FB2_in), Qp - Calculation/2(FV2_in)
  ThermalMass1/1 -> first media/2(FB1_in), Qp - Calculation/1(FV1_in)
  first media/2(Q_env) -> Sum7/1
  second media/2(Q_env) -> Sum7/2
  Sum7/1 -> Qdot_env/1
  Qp - Calculation/1(Qp_1) -> Gain/1
  Gain/1 -> first media/1(Qp)
  Qp - Calculation/2(Qp_2) -> second media/1(Qp)
  ThermalMass1/2 -> Divide1/1
  first media/1(FB1_out) -> FV1_Out/1
  second media/1(FB2_out) -> FV2_Out/1
  ThermalMass2/2 -> Divide2/1
  UA_overall/1 -> Qp - Calculation/3(UA_overall)

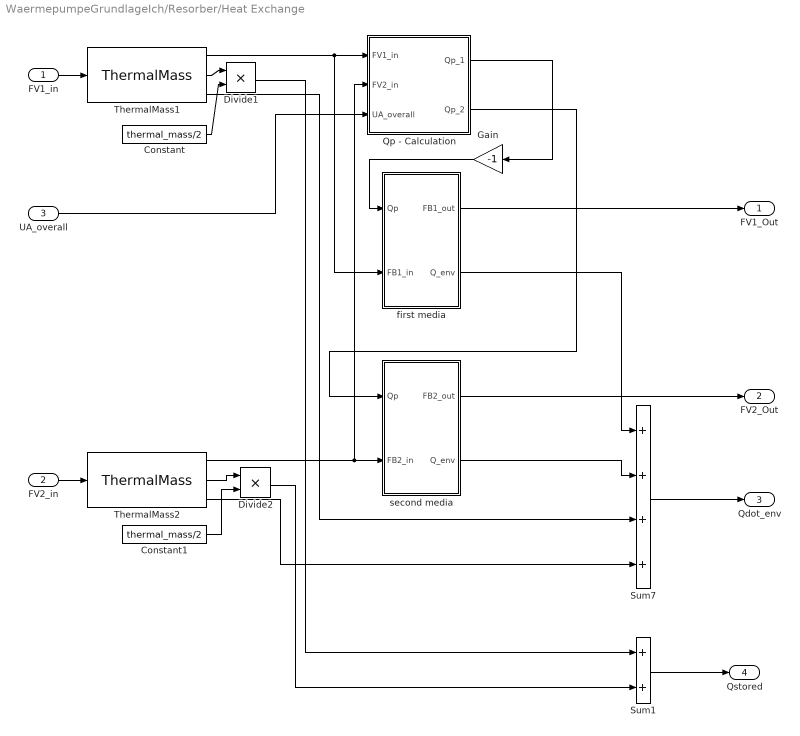
== system WaermepumpeGrundlageIch/Resorber/Heat Exchange ==
  FV1_in : Inport
  FV2_in : Inport  Port=2
  UA_overall : Inport  Port=3
  Constant : Constant  Value=thermal_mass/2
  Constant1 : Constant  Value=thermal_mass/2
  Divide1 : Product  Inputs=**
  Divide2 : Product  Inputs=**
  Gain : Gain  Gain=-1  SaturateOnIntegerOverflow=on  OutDataTypeStr=Inherit: Same as input  ParamDataTypeStr=Inherit: Same as input
  Qp - Calculation : Subsystem
  Sum1 : Sum  Inputs=2  SaturateOnIntegerOverflow=on  InputSameDT=on  OutDataTypeStr=Inherit: Same as first input
  Sum7 : Sum  Inputs=4  SaturateOnIntegerOverflow=on  InputSameDT=on  OutDataTypeStr=Inherit: Same as first input
  ThermalMass1 : Thermolib/Components/Heat and Mass Transfer/Thermal Mass/ThermalMass  A_env=A_env/4  k_env=k_env  T_env=T_env  p_loss=p_loss_1  thermal_mass=thermal_mass/2  T_initial=T_initial  UA_flow_mass=UA_flow1_mass1
  ThermalMass2 : Thermolib/Components/Heat and Mass Transfer/Thermal Mass/ThermalMass  A_env=A_env/4  k_env=k_env  T_env=T_env  p_loss=p_loss_2  thermal_mass=thermal_mass/2  T_initial=T_initial  UA_flow_mass=UA_flow2_mass2
  first media : Subsystem
  second media : Subsystem
  FV1_Out : Outport  InitialOutput=[0]
  FV2_Out : Outport  Port=2  InitialOutput=[0]
  Qdot_env : Outport  Port=3  InitialOutput=[0]
  Qstored : Outport  Port=4  InitialOutput=[0]
  wires:
  UA_overall/1 -> Qp - Calculation/3(UA_overall)
  ThermalMass2/2 -> Divide2/1
  second media/1(FB2_out) -> FV2_Out/1
  first media/1(FB1_out) -> FV1_Out/1
  ThermalMass1/2 -> Divide1/1
  Qp - Calculation/2(Qp_2) -> second media/1(Qp)
  Gain/1 -> first media/1(Qp)
  Qp - Calculation/1(Qp_1) -> Gain/1
  Sum7/1 -> Qdot_env/1
  second media/2(Q_env) -> Sum7/2
  first media/2(Q_env) -> Sum7/1
  ThermalMass1/1 -> Qp - Calculation/1(FV1_in), first media/2(FB1_in)
  ThermalMass2/1 -> Qp - Calculation/2(FV2_in), second media/2(FB2_in)
  ThermalMass2/3 -> Sum7/4
  ThermalMass1/3 -> Sum7/3
  FV1_in/1 -> ThermalMass1/1
  FV2_in/1 -> ThermalMass2/1
  Sum1/1 -> Qstored/1
  Divide1/1 -> Sum1/1
  Constant/1 -> Divide1/2
  Constant1/1 -> Divide2/2
  Divide2/1 -> Sum1/2

== system WaermepumpeGrundlageIch/Resorber/delta Hdot ==
  In1 : Inport
  In2 : Inport  Port=2
  Sensor8 : Thermolib/Miscellaneous/Sensor  lst_physical_value=Hdot measured in W;  mult_fac=1  add_fac=0  selected_signals=4
  Sensor9 : Thermolib/Miscellaneous/Sensor  lst_physical_value=Hdot measured in W;  mult_fac=1  add_fac=0  selected_signals=4
  Sum : Sum  Inputs=|+-
  Out1 : Outport
  wires:
  Sensor9/1 -> Sum/1
  Sum/1 -> Out1/1
  Sensor8/1 -> Sum/2
  In1/1 -> Sensor9/1
  In2/1 -> Sensor8/1

== system WaermepumpeGrundlageIch/Verdichter/Subsystem1 ==
  In1 : Inport
  In2 : Inport  Port=2
  In4 : Inport  Port=3
  In5 : Inport  Port=4
  Add1 : Sum
  Add4 : Sum
  Add6 : Sum
  Display11 : Display
  Display19 : Display
  Divide : Product  Inputs=*/
  Divide1 : Product  Inputs=*/
  Out1 : Outport
  tag scope: H_V=global
  wires:
  In2/1 -> Add4/2, Divide1/1, Divide/1, Add6/2
  Divide/1 -> Add1/1
  Add1/1 -> Display19/1, Out1/1
  In1/1 -> Add6/1, Add4/1
  Divide1/1 -> Display11/1
  In4/1 -> Divide/2
  Add4/1 -> Divide1/2
  In5/1 -> Add1/2
  Add6/1 -> [H_V]

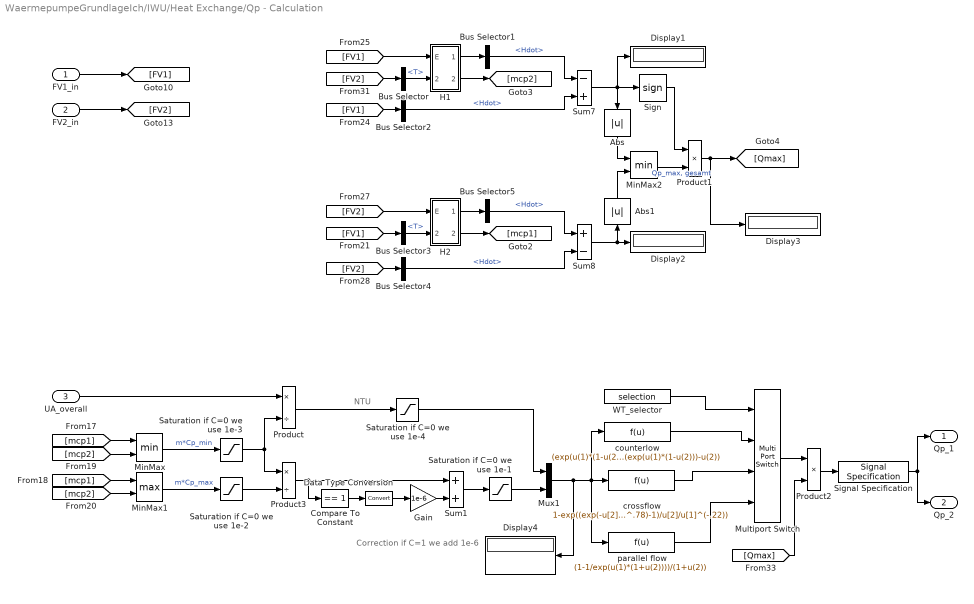
== system WaermepumpeGrundlageIch/IWU/Heat Exchange/Qp - Calculation ==
  note: Correction if C=1
      | we add 1e-6
  note: NTU
  FV1_in : Inport
  FV2_in : Inport  Port=2
  UA_overall : Inport  Port=3
  Abs : Abs
  Abs1 : Abs
  Bus Selector : BusSelector  OutputSignals=T
  Bus Selector{1..2,4..5} (4 alike) : BusSelector  OutputSignals=Hdot
  Bus Selector3 : BusSelector  OutputSignals=T
  Compare To Constant : simulink/Logic and Bit Operations/Compare To Constant  relop===  const=1  OutDataTypeStr=uint8  ZeroCross=off
  Data Type Conversion : DataTypeConversion
  Display{1..4} (4 alike) : Display
  Gain : Gain  Gain=1e-6
  H1 : Subsystem  TreatAsAtomicUnit=on  mask(H){}
      mask Display: disp('H_g')
  H2 : Subsystem  TreatAsAtomicUnit=on  mask(H){}
      mask Display: disp('H_g')
  MinMax : MinMax  Inputs=2  SaturateOnIntegerOverflow=on  InputSameDT=on
  MinMax1 : MinMax  Function=max  Inputs=2  SaturateOnIntegerOverflow=on  InputSameDT=on
  MinMax2 : MinMax  Inputs=2  SaturateOnIntegerOverflow=on  InputSameDT=on
  Multiport Switch : MultiPortSwitch  SaturateOnIntegerOverflow=on
  Mux1 : Mux  Inputs=2
  Product : Product  Inputs=*/  SaturateOnIntegerOverflow=on  InputSameDT=on  OutDataTypeStr=Inherit: Same as first input
  Product1 : Product  SaturateOnIntegerOverflow=on  InputSameDT=on  OutDataTypeStr=Inherit: Same as first input
  Product2 : Product  SaturateOnIntegerOverflow=on  InputSameDT=on  OutDataTypeStr=Inherit: Same as first input
  Product3 : Product  Inputs=*/  SaturateOnIntegerOverflow=on  InputSameDT=on  OutDataTypeStr=Inherit: Same as first input
  Saturation if C=0 we use 1e-1 : Saturate  UpperLimit=1e19  LowerLimit=1e-19
  Saturation if C=0 we use 1e-2 : Saturate  UpperLimit=1e19  LowerLimit=1e-19
  Saturation if C=0 we use 1e-3 : Saturate  UpperLimit=1e19  LowerLimit=1e-19
  Saturation if C=0 we use 1e-4 : Saturate  UpperLimit=100  LowerLimit=1e-19
  Sign : Signum
  Signal Specification : SignalSpecification  Dimensions=1
  Sum1 : Sum  Inputs=2  SaturateOnIntegerOverflow=on  InputSameDT=on  OutDataTypeStr=Inherit: Same as first input
  Sum7 : Sum  Inputs=-+  SaturateOnIntegerOverflow=on  InputSameDT=on  OutDataTypeStr=Inherit: Same as first input
  Sum8 : Sum  Inputs=+-  SaturateOnIntegerOverflow=on  InputSameDT=on  OutDataTypeStr=Inherit: Same as first input
  WT_selector : Constant  Value=selection
  counterlow : Fcn  Expr=(exp(u(1)*(1-u(2)))-1)/(exp(u(1)*(1-u(2)))-u(2))
  crossflow : Fcn  Expr=1-exp((exp(-u[2]*u[1]^.78)-1)/u[2]/u[1]^(-.22))
  parallel flow : Fcn  Expr=(1-1/exp(u(1)*(1+u(2))))/(1+u(2))
  Qp_1 : Outport
  Qp_2 : Outport  Port=2
  wires:
  Signal Specification/1 -> Qp_2/1, Qp_1/1
  Bus Selector5/1 -> Sum8/1  "<Hdot>"
  Bus Selector4/1 -> Sum8/2  "<Hdot>"
  Bus Selector2/1 -> Sum7/2  "<Hdot>"
  Bus Selector1/1 -> Sum7/1  "<Hdot>"
  Saturation if C=0 we use 1e-1/1 -> Mux1/2
  Saturation if C=0 we use 1e-3/1 -> Product/2, Product3/1
  Saturation if C=0 we use 1e-2/1 -> Product3/2
  Sum1/1 -> Saturation if C=0 we use 1e-1/1
  Gain/1 -> Sum1/2
  Data Type Conversion/1 -> Gain/1
  Compare To Constant/1 -> Data Type Conversion/1
  Product2/1 -> Signal Specification/1
  Mux1/1 -> Display4/1, counterlow/1, parallel flow/1, crossflow/1
  Product3/1 -> Sum1/1, Compare To Constant/1
  MinMax1/1 -> Saturation if C=0 we use 1e-2/1  "m*Cp_max"
  FV1_in/1 -> [FV1]
  FV2_in/1 -> [FV2]
  Product/1 -> Saturation if C=0 we use 1e-4/1
  MinMax/1 -> Saturation if C=0 we use 1e-3/1  "m*Cp_min"
  [mcp1] -> MinMax/1
  [mcp1] -> MinMax1/1
  [mcp2] -> MinMax1/2
  [mcp2] -> MinMax/2
  [Qmax] -> Product2/2
  Multiport Switch/1 -> Product2/1
  counterlow/1 -> Multiport Switch/2
  crossflow/1 -> Multiport Switch/3
  parallel flow/1 -> Multiport Switch/4
  WT_selector/1 -> Multiport Switch/1
  Bus Selector/1 -> H1/2(Temp)  "<T>"
  Bus Selector3/1 -> H2/2(Temp)  "<T>"
  [FV2] -> Bus Selector/1
  [FV2] -> Bus Selector4/1
  [FV2] -> H2/1(E)
  [FV1] -> H1/1(E)
  [FV1] -> Bus Selector2/1
  [FV1] -> Bus Selector3/1
  Sum8/1 -> Abs1/1, Display2/1
  H2/1(FB_out) -> Bus Selector5/1
  Sum7/1 -> Abs/1, Sign/1, Display1/1
  H1/1(FB_out) -> Bus Selector1/1
  MinMax2/1 -> Product1/2  "Qp_max, gesamt"
  Sign/1 -> Product1/1
  Abs/1 -> MinMax2/1
  Abs1/1 -> MinMax2/2
  Product1/1 -> [Qmax], Display3/1
  H2/2(Cp) -> [mcp1]
  H1/2(Cp) -> [mcp2]
  Saturation if C=0 we use 1e-4/1 -> Mux1/1
  UA_overall/1 -> Product/1

== system WaermepumpeGrundlageIch/IWU/Heat Exchange/first media ==
  Qp : Inport
  FB1_in : Inport  Port=2
  Bus Assignment : BusAssignment  AssignedSignals=Hdot
  Bus Selector : BusSelector  OutputSignals=Hdot
  H-p-State with HeatLoss : Thermolib/Thermodynamic States and Properties/H-p-State with Heat Exchange  k=k_env  A_total=A_env/4  T_env=T_env  relaxation_factor=0.01  conv_limit=TH_THERM_H_P_STATE_T_CONV_LIMIT  hm_conv_limit=TH_THERM_H_P_STATE_HM_CONV_LIMIT  n_iteration=TH_THERM_H_P_STATE_NUM_ITER_MAX  T_initial=T_initial  H_initial=0  ndot_zero_eps=TH_THERM_NDOT_MIN
  Sum7 : Sum  Inputs=2  SaturateOnIntegerOverflow=on  InputSameDT=on  OutDataTypeStr=Inherit: Same as first input
  Terminator4 : Terminator
  FB1_out : Outport
  Q_env : Outport  Port=2
  wires:
  Bus Assignment/1 -> H-p-State with HeatLoss/1
  H-p-State with HeatLoss/2 -> Q_env/1
  H-p-State with HeatLoss/1 -> FB1_out/1
  Bus Selector/1 -> Sum7/2  "<Hdot>"
  Sum7/1 -> Bus Assignment/2
  Qp/1 -> Sum7/1
  FB1_in/1 -> Bus Assignment/1, Bus Selector/1
  H-p-State with HeatLoss/3 -> Terminator4/1

== system WaermepumpeGrundlageIch/IWU/Heat Exchange/second media ==
  Qp : Inport
  FB2_in : Inport  Port=2
  Bus Assignment : BusAssignment  AssignedSignals=Hdot
  Bus Selector : BusSelector  OutputSignals=Hdot
  H-p-State with HeatLoss1 : Thermolib/Thermodynamic States and Properties/H-p-State with Heat Exchange  k=k_env  A_total=A_env/4  T_env=T_env  relaxation_factor=0.01  conv_limit=TH_THERM_H_P_STATE_T_CONV_LIMIT  hm_conv_limit=TH_THERM_H_P_STATE_HM_CONV_LIMIT  n_iteration=TH_THERM_H_P_STATE_NUM_ITER_MAX  T_initial=T_initial  H_initial=0  ndot_zero_eps=TH_THERM_NDOT_MIN
  Sum1 : Sum  Inputs=2  SaturateOnIntegerOverflow=on  InputSameDT=on  OutDataTypeStr=Inherit: Same as first input
  Terminator4 : Terminator
  FB2_out : Outport
  Q_env : Outport  Port=2
  wires:
  Bus Selector/1 -> Sum1/2  "<Hdot>"
  Bus Assignment/1 -> H-p-State with HeatLoss1/1
  H-p-State with HeatLoss1/2 -> Q_env/1
  FB2_in/1 -> Bus Assignment/1, Bus Selector/1
  Qp/1 -> Sum1/1
  Sum1/1 -> Bus Assignment/2
  H-p-State with HeatLoss1/1 -> FB2_out/1
  H-p-State with HeatLoss1/3 -> Terminator4/1

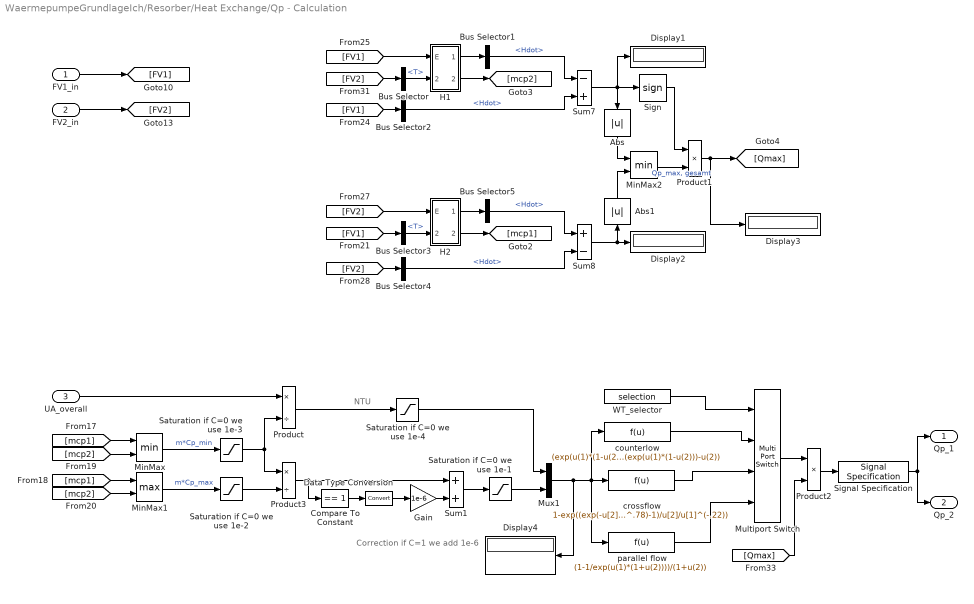
== system WaermepumpeGrundlageIch/Resorber/Heat Exchange/Qp - Calculation ==
  note: NTU
  note: Correction if C=1
      | we add 1e-6
  FV1_in : Inport
  FV2_in : Inport  Port=2
  UA_overall : Inport  Port=3
  Abs : Abs
  Abs1 : Abs
  Bus Selector : BusSelector  OutputSignals=T
  Bus Selector{1..2,4..5} (4 alike) : BusSelector  OutputSignals=Hdot
  Bus Selector3 : BusSelector  OutputSignals=T
  Compare To Constant : simulink/Logic and Bit Operations/Compare To Constant  relop===  const=1  OutDataTypeStr=uint8  ZeroCross=off
  Data Type Conversion : DataTypeConversion
  Display{1..4} (4 alike) : Display
  Gain : Gain  Gain=1e-6
  H1 : Subsystem  TreatAsAtomicUnit=on  mask(H){}
      mask Display: disp('H_g')
  H2 : Subsystem  TreatAsAtomicUnit=on  mask(H){}
      mask Display: disp('H_g')
  MinMax : MinMax  Inputs=2  SaturateOnIntegerOverflow=on  InputSameDT=on
  MinMax1 : MinMax  Function=max  Inputs=2  SaturateOnIntegerOverflow=on  InputSameDT=on
  MinMax2 : MinMax  Inputs=2  SaturateOnIntegerOverflow=on  InputSameDT=on
  Multiport Switch : MultiPortSwitch  SaturateOnIntegerOverflow=on
  Mux1 : Mux  Inputs=2
  Product : Product  Inputs=*/  SaturateOnIntegerOverflow=on  InputSameDT=on  OutDataTypeStr=Inherit: Same as first input
  Product1 : Product  SaturateOnIntegerOverflow=on  InputSameDT=on  OutDataTypeStr=Inherit: Same as first input
  Product2 : Product  SaturateOnIntegerOverflow=on  InputSameDT=on  OutDataTypeStr=Inherit: Same as first input
  Product3 : Product  Inputs=*/  SaturateOnIntegerOverflow=on  InputSameDT=on  OutDataTypeStr=Inherit: Same as first input
  Saturation if C=0 we use 1e-1 : Saturate  UpperLimit=1e19  LowerLimit=1e-19
  Saturation if C=0 we use 1e-2 : Saturate  UpperLimit=1e19  LowerLimit=1e-19
  Saturation if C=0 we use 1e-3 : Saturate  UpperLimit=1e19  LowerLimit=1e-19
  Saturation if C=0 we use 1e-4 : Saturate  UpperLimit=100  LowerLimit=1e-19
  Sign : Signum
  Signal Specification : SignalSpecification  Dimensions=1
  Sum1 : Sum  Inputs=2  SaturateOnIntegerOverflow=on  InputSameDT=on  OutDataTypeStr=Inherit: Same as first input
  Sum7 : Sum  Inputs=-+  SaturateOnIntegerOverflow=on  InputSameDT=on  OutDataTypeStr=Inherit: Same as first input
  Sum8 : Sum  Inputs=+-  SaturateOnIntegerOverflow=on  InputSameDT=on  OutDataTypeStr=Inherit: Same as first input
  WT_selector : Constant  Value=selection
  counterlow : Fcn  Expr=(exp(u(1)*(1-u(2)))-1)/(exp(u(1)*(1-u(2)))-u(2))
  crossflow : Fcn  Expr=1-exp((exp(-u[2]*u[1]^.78)-1)/u[2]/u[1]^(-.22))
  parallel flow : Fcn  Expr=(1-1/exp(u(1)*(1+u(2))))/(1+u(2))
  Qp_1 : Outport
  Qp_2 : Outport  Port=2
  wires:
  UA_overall/1 -> Product/1
  Saturation if C=0 we use 1e-4/1 -> Mux1/1
  H1/2(Cp) -> [mcp2]
  H2/2(Cp) -> [mcp1]
  Product1/1 -> Display3/1, [Qmax]
  Abs1/1 -> MinMax2/2
  Abs/1 -> MinMax2/1
  Sign/1 -> Product1/1
  MinMax2/1 -> Product1/2  "Qp_max, gesamt"
  H1/1(FB_out) -> Bus Selector1/1
  Sum7/1 -> Display1/1, Sign/1, Abs/1
  H2/1(FB_out) -> Bus Selector5/1
  Sum8/1 -> Display2/1, Abs1/1
  [FV1] -> Bus Selector3/1
  [FV1] -> Bus Selector2/1
  [FV1] -> H1/1(E)
  [FV2] -> H2/1(E)
  [FV2] -> Bus Selector4/1
  [FV2] -> Bus Selector/1
  Bus Selector3/1 -> H2/2(Temp)  "<T>"
  Bus Selector/1 -> H1/2(Temp)  "<T>"
  WT_selector/1 -> Multiport Switch/1
  parallel flow/1 -> Multiport Switch/4
  crossflow/1 -> Multiport Switch/3
  counterlow/1 -> Multiport Switch/2
  Multiport Switch/1 -> Product2/1
  [Qmax] -> Product2/2
  [mcp2] -> MinMax/2
  [mcp2] -> MinMax1/2
  [mcp1] -> MinMax1/1
  [mcp1] -> MinMax/1
  MinMax/1 -> Saturation if C=0 we use 1e-3/1  "m*Cp_min"
  Product/1 -> Saturation if C=0 we use 1e-4/1
  FV2_in/1 -> [FV2]
  FV1_in/1 -> [FV1]
  MinMax1/1 -> Saturation if C=0 we use 1e-2/1  "m*Cp_max"
  Product3/1 -> Compare To Constant/1, Sum1/1
  Mux1/1 -> crossflow/1, parallel flow/1, counterlow/1, Display4/1
  Product2/1 -> Signal Specification/1
  Compare To Constant/1 -> Data Type Conversion/1
  Data Type Conversion/1 -> Gain/1
  Gain/1 -> Sum1/2
  Sum1/1 -> Saturation if C=0 we use 1e-1/1
  Saturation if C=0 we use 1e-2/1 -> Product3/2
  Saturation if C=0 we use 1e-3/1 -> Product3/1, Product/2
  Saturation if C=0 we use 1e-1/1 -> Mux1/2
  Bus Selector1/1 -> Sum7/1  "<Hdot>"
  Bus Selector2/1 -> Sum7/2  "<Hdot>"
  Bus Selector4/1 -> Sum8/2  "<Hdot>"
  Bus Selector5/1 -> Sum8/1  "<Hdot>"
  Signal Specification/1 -> Qp_1/1, Qp_2/1
